simulink model "TFlex_FRF"  (R2018a)
settings: Solver=FixedStepDiscrete  StartTime=0.0  StopTime=t_end  FixedStep=0.001  RelTol=1e-3
PreLoadFcn:
  | Ts = 0.001;
InitFcn:
  | Ts = 0.001;
values from neighbouring files (symbols this model uses):
  t_end = 200    [Tflex_PID_init.m]    (also in multisineInit.m = t(end))
  ts = 1/1000    (= 0.001)    [Tflex_PID_init.m]    (also in init.m = 0.00025; multisineInit.m)
libraries: xpcethercatlib x91, simulink x60, slrtlib x6
(part 1 of 2)
settings Model: xpc_rtwmakecfg_data=_xpcethercatlib_  SimulationMode=external  ExtModeTrigDirection=either  ExplicitPartitioning=on  Creator=lab  LastModifiedBy=wout7
settings DataIOCC: Decimation=10  LimitDataPoints=on  SaveFormat=StructureWithTime
settings OptimizationCC: BlockReduction=off  OptimizeBlockIOStorage=off  BufferReuse=off  GlobalBufferReuse=off  ExpressionFolding=off  LocalBlockOutputs=off  OptimizeDataStoreBuffers=off  BusAssignmentInplaceUpdate=off
settings DebuggingCC: UnconnectedInputMsg=none  UnconnectedOutputMsg=none  UnconnectedLineMsg=none
settings HardwareCC: ProdBitPerPointer=32  ProdBitPerSizeT=32  ProdBitPerPtrDiffT=32  ProdLargestAtomicFloat=None  ProdWordSize=32  ProdLongLongMode=on  ProdHWDeviceType=Generic->32-bit x86 compatible
settings RTWCC: SystemTargetFile=slrt.tlc  TemplateMakefile=slrt_default_tmf  Description=Simulink Real-Time  CodeExecutionProfiling=on
settings SimulinkRealTimeCC: SupportVariableSizeSignals=on  xPCConcurrentTasks=on

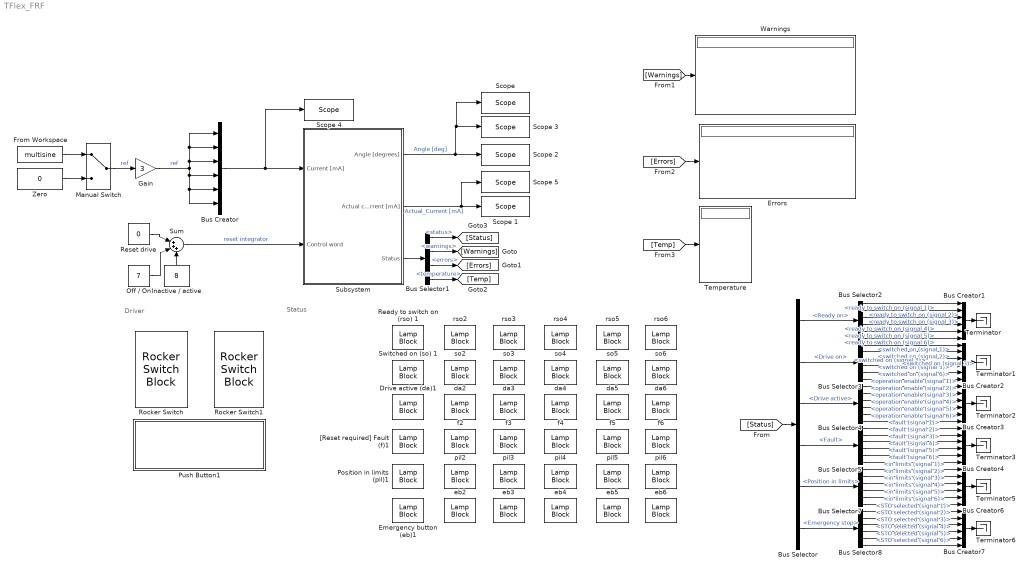
== system TFlex_FRF ==
  note: Driver
  note: Status
  " da2 " : LampBlock  WebBlockId=1372  LabelPosition=Hide
  " so2 " : LampBlock  WebBlockId=1336  LabelPosition=Hide
  " da4" : LampBlock  WebBlockId=1373  LabelPosition=Hide
  " da5" : LampBlock  WebBlockId=1374  LabelPosition=Hide
  " da6" : LampBlock  WebBlockId=1375  LabelPosition=Hide
  " eb4" : LampBlock  WebBlockId=1402  LabelPosition=Hide
  " eb5" : LampBlock  WebBlockId=1403  LabelPosition=Hide
  " eb6" : LampBlock  WebBlockId=1404  LabelPosition=Hide
  " f4" : LampBlock  WebBlockId=1379  LabelPosition=Hide
  " f5" : LampBlock  WebBlockId=1380  LabelPosition=Hide
  " f6" : LampBlock  WebBlockId=1381  LabelPosition=Hide
  " pil4" : LampBlock  WebBlockId=1397  LabelPosition=Hide
  " pil5" : LampBlock  WebBlockId=1398  LabelPosition=Hide
  " pil6" : LampBlock  WebBlockId=1399  LabelPosition=Hide
  " rso4" : LampBlock  WebBlockId=1325  LabelPosition=Hide
  " so4" : LampBlock  WebBlockId=1333  LabelPosition=Hide
  " so5" : LampBlock  WebBlockId=1334  LabelPosition=Hide
  " so6" : LampBlock  WebBlockId=1335  LabelPosition=Hide
  Bus Creator{,1..4,6..7} (7 alike) : BusCreator  Inputs=6
  Bus Selector : BusSelector  OutputSignals=Ready on,Drive on,Drive active,Fault,Position in limits,Emergency stop
  Bus Selector1 : BusSelector  OutputSignals=status,warnings,errors,temperature
  Bus Selector2 : BusSelector  OutputSignals=ready to switch on (signal 1),ready to switch on (signal 2),ready to switch on (signal 3),ready to switch on (signal 4),ready to switch on (signal 5),ready to switch on (signal 6)
  Bus Selector3 : BusSelector  OutputSignals=switched on (signal 1),switched on (signal 2),switched on (signal 3),switched on (signal 4),switched on (signal 5),switched on (signal 6)
  Bus Selector4 : BusSelector  OutputSignals=operation enable (signal 1),operation enable (signal 2),operation enable (signal 3),operation enable (signal 4),operation enable (signal 5),operation enable (signal 6)
  Bus Selector5 : BusSelector  OutputSignals=fault (signal 1),fault (signal 2),fault (signal 3),fault (signal 4),fault (signal 5),fault (signal 6)
  Bus Selector7 : BusSelector  OutputSignals=in limits (signal 1),in limits (signal 2),in limits (signal 3),in limits (signal 4),in limits (signal 5),in limits (signal 6)
  Bus Selector8 : BusSelector  OutputSignals=STO selected (signal 1),STO selected (signal 2),STO selected (signal 3),STO selected (signal 4),STO selected (signal 5),STO selected (signal 6)
  Drive active (da)1 : LampBlock  WebBlockId=1376
  Emergency button (eb)1 : LampBlock  WebBlockId=1405
  Errors : Display
      settings: Decimation=25
  From Workspace : FromWorkspace  VariableName=multisine  OutputAfterFinalValue=Setting to zero
  Gain : Gain  Gain=3
  Inactive / active : Constant  Value=8  SampleTime=-1
  Manual Switch : ManualSwitch
  Off / On : Constant  Value=7  SampleTime=-1
  Position in limits (pil)1 : LampBlock  WebBlockId=1400
  Push Button1 : Subsystem  DialogController=hmiCreateDDGDialog  IsWebBlock=on  mask(MWDashboardBlock){webBlockId=c834c18b-4d14-4fd2-a2aa-8470ccae1b8a, webBlockType=pushbutton, ShowInLibBrwoser=on, ShowInitialText=on, HMISrcModelName=TFlex_FRF}
      mask prompts: webBlockId "WebBlock Id"; webBlockType "WebBlock Type"; HMISrcModelName "Source Model"
      mask help: SimulinkHMI:dialogs:PushButtonDialogDesc
      mask Help: helpview([docroot '/mapfiles/simulink.map'], 'hmi_push_button')
      mask Display:
      | model = bdroot(gcb);
      | if strcmp(get_param(model,'BlockDiagramType'), 'library')
      |     image([(matlabroot) '/toolbox/simulink/hmi/icons/PushButton.png']);
      | end
  Ready to switch on (rso) 1 : LampBlock  WebBlockId=226
  Reset drive : Constant  Value=0  SampleTime=-1
  Rocker Switch : RockerSwitchBlock  WebBlockId=231
      settings: Values={{'Off', 'On'}, [6 7]}
  Rocker Switch1 : RockerSwitchBlock  WebBlockId=232
      settings: Values={{'Off', 'On'}, [0 8]}
  "Scope " : slrtlib/Displays and Logging/Scope   scopeno=4  scopetype=File  autostart=on  viewmode=Graphical redraw  formatstr='%15.6f'  grid=on  ylimits=[0,0]  nosamples=t_end/ts  noprepostsamples=0  interleave=1  triggermode=FreeRun  triggersignal=1  trigsignalfromport=off  triggerlevel=0.0  triggerslope=Either  triggerscope=1  triggersample=0  filename=ANGLE.dat  mode=Lazy  writesize=512  autorestart=off  dynamicfilemode=off  maxwritefilesize=512*1024^2
  Scope 1 : slrtlib/Displays and Logging/Scope   scopeno=2  scopetype=Target  autostart=on  viewmode=Graphical sliding  formatstr='%15.6f,%15.6f,%15.6f,%15.6f,%15.6f,%15.6f'  grid=on  ylimits=[-500,500]  nosamples=2000  noprepostsamples=0  interleave=25  triggermode=FreeRun  triggersignal=1  trigsignalfromport=off  triggerlevel=0.0  triggerslope=Either  triggerscope=1  triggersample=0  filename=data.dat  mode=Lazy  writesize=512  autorestart=off  dynamicfilemode=off  maxwritefilesize=512*1024^2
  Scope 2 : slrtlib/Displays and Logging/Scope   scopeno=1  scopetype=Target  autostart=on  viewmode=Numerical  formatstr='%15.6f,%15.6f,%15.6f,%15.6f,%15.6f,%15.6f'  grid=on  ylimits=[500,500]  nosamples=100  noprepostsamples=0  interleave=25  triggermode=FreeRun  triggersignal=1  trigsignalfromport=off  triggerlevel=0.0  triggerslope=Either  triggerscope=1  triggersample=0  filename=data.dat  mode=Lazy  writesize=512  autorestart=off  dynamicfilemode=off  maxwritefilesize=512*1024^2
  Scope 3 : slrtlib/Displays and Logging/Scope   scopeno=3  scopetype=Target  autostart=on  viewmode=Graphical sliding  formatstr='%15.6f,%15.6f,%15.6f,%15.6f,%15.6f,%15.6f'  grid=on  ylimits=[-20,20]  nosamples=3000  noprepostsamples=0  interleave=25  triggermode=FreeRun  triggersignal=1  trigsignalfromport=off  triggerlevel=0.0  triggerslope=Either  triggerscope=1  triggersample=0  filename=data.dat  mode=Lazy  writesize=512  autorestart=off  dynamicfilemode=off  maxwritefilesize=512*1024^2
  Scope 4 : slrtlib/Displays and Logging/Scope   scopeno=5  scopetype=File  autostart=on  viewmode=Graphical redraw  formatstr='%15.6f'  grid=on  ylimits=[0,0]  nosamples=t_end/ts  noprepostsamples=0  interleave=1  triggermode=FreeRun  triggersignal=1  trigsignalfromport=off  triggerlevel=0.0  triggerslope=Either  triggerscope=1  triggersample=0  filename=I_SP.dat  mode=Lazy  writesize=512  autorestart=off  dynamicfilemode=off  maxwritefilesize=512*1024^2
  Scope 5 : slrtlib/Displays and Logging/Scope   scopeno=6  scopetype=File  autostart=on  viewmode=Graphical redraw  formatstr='%15.6f'  grid=on  ylimits=[0,0]  nosamples=t_end/ts  noprepostsamples=0  interleave=1  triggermode=FreeRun  triggersignal=1  trigsignalfromport=off  triggerlevel=0.0  triggerslope=Either  triggerscope=1  triggersample=0  filename=I_A.dat  mode=Lazy  writesize=512  autorestart=off  dynamicfilemode=off  maxwritefilesize=512*1024^2
  Subsystem : Subsystem  TreatAsAtomicUnit=on
  Sum : Sum  Inputs=|+++
  Switched on (so) 1 : LampBlock  WebBlockId=1338
  Temperature : Display
      settings: Decimation=25
  Terminator{,1..3,5..6} (6 alike) : Terminator
  Warnings : Display
      settings: Decimation=25
  Zero : Constant  Value=0
  "[Reset required] Fault (f)1 " : LampBlock  WebBlockId=1382
  da3 : LampBlock  WebBlockId=1377  LabelPosition=Hide
  eb2 : LampBlock  WebBlockId=1406  LabelPosition=Hide
  eb3 : LampBlock  WebBlockId=1407  LabelPosition=Hide
  f2 : LampBlock  WebBlockId=1378  LabelPosition=Hide
  f3 : LampBlock  WebBlockId=1383  LabelPosition=Hide
  pil2 : LampBlock  WebBlockId=1396  LabelPosition=Hide
  pil3 : LampBlock  WebBlockId=1401  LabelPosition=Hide
  rso2 : LampBlock  WebBlockId=1323  LabelPosition=Hide
  rso3 : LampBlock  WebBlockId=1324  LabelPosition=Hide
  rso5 : LampBlock  WebBlockId=1326  LabelPosition=Hide
  rso6 : LampBlock  WebBlockId=1327  LabelPosition=Hide
  so3 : LampBlock  WebBlockId=1337  LabelPosition=Hide
  wires:
  Subsystem/2(Actual current [mA]) -> Scope 5/1, Scope 1/1  "Actual_Current [mA]"
  Bus Selector/1 -> Bus Selector2/1  "<Ready on>"
  Bus Selector/2 -> Bus Selector3/1  "<Drive on>"
  Bus Selector/3 -> Bus Selector4/1  "<Drive active>"
  Bus Selector/4 -> Bus Selector5/1  "<Fault>"
  Bus Selector/5 -> Bus Selector7/1  "<Position in limits>"
  Bus Selector/6 -> Bus Selector8/1  "<Emergency stop>"
  Reset drive/1 -> Sum/1
  Off / On/1 -> Sum/2
  Inactive / active/1 -> Sum/3
  Subsystem/1(Angle [degrees]) -> "Scope "/1, Scope 3/1, Scope 2/1  "Angle [deg]"
  Manual Switch/1 -> Gain/1  "ref"
  Subsystem/3(Status) -> Bus Selector1/1
  [Temp] -> Temperature/1
  [Errors] -> Errors/1
  [Warnings] -> Warnings/1
  [Status] -> Bus Selector/1
  Bus Selector2/1 -> Bus Creator1/1  "<ready to switch on (signal 1)>"
  Bus Selector2/2 -> Bus Creator1/2  "<ready to switch on (signal 2)>"
  Bus Selector2/3 -> Bus Creator1/3  "<ready to switch on (signal 3)>"
  Bus Selector2/4 -> Bus Creator1/4  "<ready to switch on (signal 4)>"
  Bus Selector2/5 -> Bus Creator1/5  "<ready to switch on (signal 5)>"
  Bus Selector2/6 -> Bus Creator1/6  "<ready to switch on (signal 6)>"
  Bus Creator1/1 -> Terminator/1
  Bus Selector3/2 -> Bus Creator2/2  "<switched on (signal 2)>"
  Bus Selector3/1 -> Bus Creator2/1  "<switched on (signal 1)>"
  Bus Selector3/5 -> Bus Creator2/5  "<switched on (signal 5)>"
  Bus Creator2/1 -> Terminator1/1
  Bus Selector3/4 -> Bus Creator2/4  "<switched on (signal 4)>"
  Bus Selector3/6 -> Bus Creator2/6  "<switched on (signal 6)>"
  Bus Selector3/3 -> Bus Creator2/3  "<switched on (signal 3)>"
  Bus Selector4/4 -> Bus Creator3/4  "<operation enable (signal 4)>"
  Bus Selector4/6 -> Bus Creator3/6  "<operation enable (signal 6)>"
  Bus Creator3/1 -> Terminator2/1
  Bus Selector4/5 -> Bus Creator3/5  "<operation enable (signal 5)>"
  Bus Selector4/1 -> Bus Creator3/1  "<operation enable (signal 1)>"
  Bus Selector4/2 -> Bus Creator3/2  "<operation enable (signal 2)>"
  Bus Selector4/3 -> Bus Creator3/3  "<operation enable (signal 3)>"
  Bus Selector5/4 -> Bus Creator4/4  "<fault (signal 4)>"
  Bus Selector5/6 -> Bus Creator4/6  "<fault (signal 6)>"
  Bus Creator4/1 -> Terminator3/1
  Bus Selector5/5 -> Bus Creator4/5  "<fault (signal 5)>"
  Bus Selector5/1 -> Bus Creator4/1  "<fault (signal 1)>"
  Bus Selector5/2 -> Bus Creator4/2  "<fault (signal 2)>"
  Bus Selector5/3 -> Bus Creator4/3  "<fault (signal 3)>"
  Bus Selector7/4 -> Bus Creator6/4  "<in limits (signal 4)>"
  Bus Selector7/6 -> Bus Creator6/6  "<in limits (signal 6)>"
  Bus Creator6/1 -> Terminator5/1
  Bus Selector7/5 -> Bus Creator6/5  "<in limits (signal 5)>"
  Bus Selector7/1 -> Bus Creator6/1  "<in limits (signal 1)>"
  Bus Selector7/2 -> Bus Creator6/2  "<in limits (signal 2)>"
  Bus Selector7/3 -> Bus Creator6/3  "<in limits (signal 3)>"
  Bus Selector8/4 -> Bus Creator7/4  "<STO selected (signal 4)>"
  Bus Selector8/6 -> Bus Creator7/6  "<STO selected (signal 6)>"
  Bus Creator7/1 -> Terminator6/1
  Bus Selector8/5 -> Bus Creator7/5  "<STO selected (signal 5)>"
  Bus Selector8/1 -> Bus Creator7/1  "<STO selected (signal 1)>"
  Bus Selector8/2 -> Bus Creator7/2  "<STO selected (signal 2)>"
  Bus Selector8/3 -> Bus Creator7/3  "<STO selected (signal 3)>"
  Bus Creator/1 -> Scope 4/1, Subsystem/1(Current [mA])
  Sum/1 -> Subsystem/2(Control word)  "reset integrator"
  Bus Selector1/1 -> [Status]  "<status>"
  Bus Selector1/2 -> [Warnings]  "<warnings>"
  Bus Selector1/3 -> [Errors]  "<errors>"
  Bus Selector1/4 -> [Temp]  "<temperature>"
  From Workspace/1 -> Manual Switch/1
  Zero/1 -> Manual Switch/2
  Gain/1 -> Bus Creator/4, Bus Creator/5, Bus Creator/6, Bus Creator/3, Bus Creator/2, Bus Creator/1  "ref"

== system TFlex_FRF/Push Button1 ==

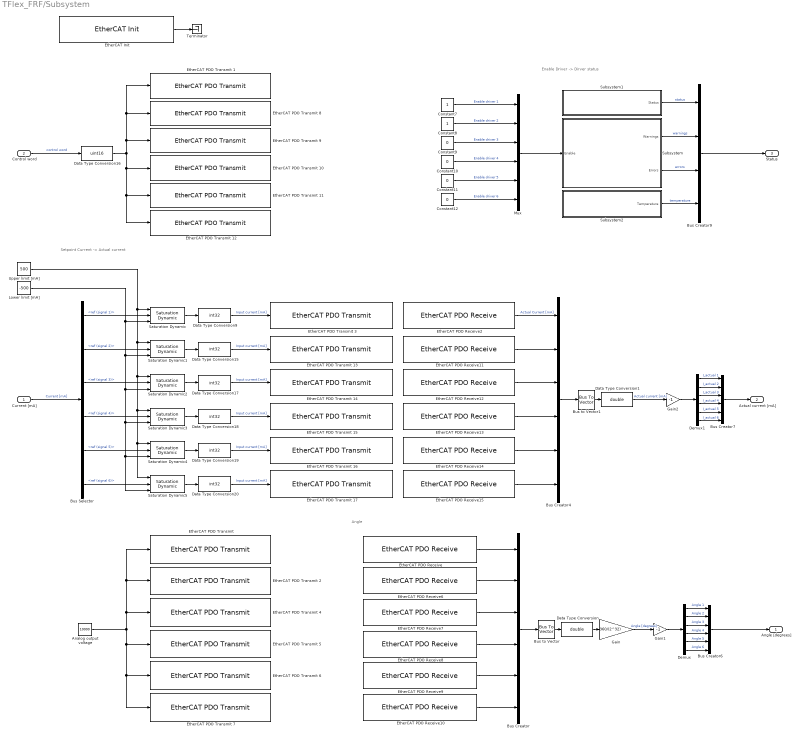
== system TFlex_FRF/Subsystem ==
  note: Angle
  note: Enable Driver -> Dirver status
  note: Setpoint Current -> Actual current
  Current [mA] : Inport  PortDimensions=6
  Control word : Inport  Port=2
  Analog output voltage : Constant  Value=10000  OutDataTypeStr=int16  SampleTime=-1
  Bus Creator{,4,6..7} (4 alike) : BusCreator  Inputs=6
  Bus Creator9 : BusCreator  Inputs=4
  Bus Selector : BusSelector  OutputSignals=ref (signal 1),ref (signal 2),ref (signal 3),ref (signal 4),ref (signal 5),ref (signal 6)
  Bus to Vector : BusToVector
  Bus to Vector1 : BusToVector
  Constant{9..12} (4 alike) : Constant  Value=0  OutDataTypeStr=int32  SampleTime=1
  Constant7 : Constant  OutDataTypeStr=int32  SampleTime=1
  Constant8 : Constant  OutDataTypeStr=int32  SampleTime=1
  Data Type Conversion : DataTypeConversion  OutDataTypeStr=double
  Data Type Conversion1 : DataTypeConversion  OutDataTypeStr=double
  Data Type Conversion{9,15,17..20} (6 alike) : DataTypeConversion  OutDataTypeStr=int32
  Data Type Conversion16 : DataTypeConversion  OutDataTypeStr=uint16
  Demux : Demux  Outputs=6
  Demux1 : Demux  Outputs=6
  "EtherCAT Init " : xpcethercatlib/EtherCAT Init   Priority=0  config_file=C:\Users\wout7\Documents\GitHub\Inverse_dynamics_learning\TargetPC\6 DOF\pdo_mapping_6dr_1kHz.xml  device_id=0  pci_bus=13  pci_slot=0  pci_function=0  dctuning=0  enaDebug=off  enaDC=on  errLink=off  masterDbg=off  stateChgDbg=off  baseClock=off  masterCfg=off  logFile='c:\dbglog.txt'  sample_time=0.001000  DCMode=2
      settings: SourceProductName=Simulink Real-Time  SourceProductBaseCode=XP
  EtherCAT PDO Receive : xpcethercatlib/EtherCAT PDO Receive  Priority=2  sig_name=Drive 2 (AKD).Inputs_1.Position actual internal value  sig_offset=560  sig_type=int32  type_size=32  sig_dim=1  device_id=0  sample_time=0.001000
      settings: SourceProductName=Simulink Real-Time  SourceProductBaseCode=XP
  EtherCAT PDO Receive10 : xpcethercatlib/EtherCAT PDO Receive  Priority=2  sig_name=Drive 7 (AKD).Inputs_1.Position actual internal value  sig_offset=37488  sig_type=int32  type_size=32  sig_dim=1  device_id=0  sample_time=0.001000
      settings: SourceProductName=Simulink Real-Time  SourceProductBaseCode=XP
  EtherCAT PDO Receive11 : xpcethercatlib/EtherCAT PDO Receive  Priority=2  sig_name=Drive 3 (AKD).Inputs_1.Current actual value  sig_offset=12560  sig_type=int32  type_size=32  sig_dim=1  device_id=0  sample_time=0.001000
      settings: SourceProductName=Simulink Real-Time  SourceProductBaseCode=XP
  EtherCAT PDO Receive12 : xpcethercatlib/EtherCAT PDO Receive  Priority=2  sig_name=Drive 4 (AKD).Inputs_1.Current actual value  sig_offset=24848  sig_type=int32  type_size=32  sig_dim=1  device_id=0  sample_time=0.001000
      settings: SourceProductName=Simulink Real-Time  SourceProductBaseCode=XP
  EtherCAT PDO Receive13 : xpcethercatlib/EtherCAT PDO Receive  Priority=2  sig_name=Drive 5 (AKD).Inputs_1.Current actual value  sig_offset=37136  sig_type=int32  type_size=32  sig_dim=1  device_id=0  sample_time=0.001000
      settings: SourceProductName=Simulink Real-Time  SourceProductBaseCode=XP
  EtherCAT PDO Receive14 : xpcethercatlib/EtherCAT PDO Receive  Priority=2  sig_name=Drive 6 (AKD).Inputs_1.Current actual value  sig_offset=37296  sig_type=int32  type_size=32  sig_dim=1  device_id=0  sample_time=0.001000
      settings: SourceProductName=Simulink Real-Time  SourceProductBaseCode=XP
  EtherCAT PDO Receive15 : xpcethercatlib/EtherCAT PDO Receive  Priority=2  sig_name=Drive 7 (AKD).Inputs_1.Current actual value  sig_offset=37456  sig_type=int32  type_size=32  sig_dim=1  device_id=0  sample_time=0.001000
      settings: SourceProductName=Simulink Real-Time  SourceProductBaseCode=XP
  EtherCAT PDO Receive2 : xpcethercatlib/EtherCAT PDO Receive  Priority=2  sig_name=Drive 2 (AKD).Inputs_1.Current actual value  sig_offset=528  sig_type=int32  type_size=32  sig_dim=1  device_id=0  sample_time=0.001000
      settings: SourceProductName=Simulink Real-Time  SourceProductBaseCode=XP
  EtherCAT PDO Receive6 : xpcethercatlib/EtherCAT PDO Receive  Priority=2  sig_name=Drive 3 (AKD).Inputs_1.Position actual internal value  sig_offset=12592  sig_type=int32  type_size=32  sig_dim=1  device_id=0  sample_time=0.001000
      settings: SourceProductName=Simulink Real-Time  SourceProductBaseCode=XP
  EtherCAT PDO Receive7 : xpcethercatlib/EtherCAT PDO Receive  Priority=2  sig_name=Drive 4 (AKD).Inputs_1.Position actual internal value  sig_offset=24880  sig_type=int32  type_size=32  sig_dim=1  device_id=0  sample_time=0.001000
      settings: SourceProductName=Simulink Real-Time  SourceProductBaseCode=XP
  EtherCAT PDO Receive8 : xpcethercatlib/EtherCAT PDO Receive  Priority=2  sig_name=Drive 5 (AKD).Inputs_1.Position actual internal value  sig_offset=37168  sig_type=int32  type_size=32  sig_dim=1  device_id=0  sample_time=0.001000
      settings: SourceProductName=Simulink Real-Time  SourceProductBaseCode=XP
  EtherCAT PDO Receive9 : xpcethercatlib/EtherCAT PDO Receive  Priority=2  sig_name=Drive 6 (AKD).Inputs_1.Position actual internal value  sig_offset=37328  sig_type=int32  type_size=32  sig_dim=1  device_id=0  sample_time=0.001000
      settings: SourceProductName=Simulink Real-Time  SourceProductBaseCode=XP
  "EtherCAT PDO Transmit " : xpcethercatlib/EtherCAT PDO Transmit   Priority=3  sig_name=Drive 2 (AKD).Outputs.AOUT.VALUE write  sig_offset=480  sig_type=int16  type_size=16  sig_dim=1  device_id=0  sample_time=0.001000
      settings: SourceProductName=Simulink Real-Time  SourceProductBaseCode=XP
  EtherCAT PDO Transmit 1 : xpcethercatlib/EtherCAT PDO Transmit   Priority=3  sig_name=Drive 2 (AKD).Outputs.Controlword  sig_offset=464  sig_type=uint16  type_size=16  sig_dim=1  device_id=0  sample_time=0.001000
      settings: SourceProductName=Simulink Real-Time  SourceProductBaseCode=XP
  EtherCAT PDO Transmit 10 : xpcethercatlib/EtherCAT PDO Transmit   Priority=3  sig_name=Drive 5 (AKD).Outputs.Controlword  sig_offset=37072  sig_type=uint16  type_size=16  sig_dim=1  device_id=0  sample_time=0.001000
      settings: SourceProductName=Simulink Real-Time  SourceProductBaseCode=XP
  EtherCAT PDO Transmit 11 : xpcethercatlib/EtherCAT PDO Transmit   Priority=3  sig_name=Drive 6 (AKD).Outputs.Controlword  sig_offset=37232  sig_type=uint16  type_size=16  sig_dim=1  device_id=0  sample_time=0.001000
      settings: SourceProductName=Simulink Real-Time  SourceProductBaseCode=XP
  EtherCAT PDO Transmit 12 : xpcethercatlib/EtherCAT PDO Transmit   Priority=3  sig_name=Drive 7 (AKD).Outputs.Controlword  sig_offset=37392  sig_type=uint16  type_size=16  sig_dim=1  device_id=0  sample_time=0.001000
      settings: SourceProductName=Simulink Real-Time  SourceProductBaseCode=XP
  EtherCAT PDO Transmit 13 : xpcethercatlib/EtherCAT PDO Transmit   Priority=3  sig_name=Drive 3 (AKD).Outputs.Target current  sig_offset=12528  sig_type=int32  type_size=32  sig_dim=1  device_id=0  sample_time=0.001000
      settings: SourceProductName=Simulink Real-Time  SourceProductBaseCode=XP
  EtherCAT PDO Transmit 14 : xpcethercatlib/EtherCAT PDO Transmit   Priority=3  sig_name=Drive 4 (AKD).Outputs.Target current  sig_offset=24816  sig_type=int32  type_size=32  sig_dim=1  device_id=0  sample_time=0.001000
      settings: SourceProductName=Simulink Real-Time  SourceProductBaseCode=XP
  EtherCAT PDO Transmit 15 : xpcethercatlib/EtherCAT PDO Transmit   Priority=3  sig_name=Drive 5 (AKD).Outputs.Target current  sig_offset=37104  sig_type=int32  type_size=32  sig_dim=1  device_id=0  sample_time=0.001000
      settings: SourceProductName=Simulink Real-Time  SourceProductBaseCode=XP
  EtherCAT PDO Transmit 16 : xpcethercatlib/EtherCAT PDO Transmit   Priority=3  sig_name=Drive 6 (AKD).Outputs.Target current  sig_offset=37264  sig_type=int32  type_size=32  sig_dim=1  device_id=0  sample_time=0.001000
      settings: SourceProductName=Simulink Real-Time  SourceProductBaseCode=XP
  EtherCAT PDO Transmit 17 : xpcethercatlib/EtherCAT PDO Transmit   Priority=3  sig_name=Drive 7 (AKD).Outputs.Target current  sig_offset=37424  sig_type=int32  type_size=32  sig_dim=1  device_id=0  sample_time=0.001000
      settings: SourceProductName=Simulink Real-Time  SourceProductBaseCode=XP
  EtherCAT PDO Transmit 2 : xpcethercatlib/EtherCAT PDO Transmit   Priority=3  sig_name=Drive 3 (AKD).Outputs.AOUT.VALUE write  sig_offset=12512  sig_type=int16  type_size=16  sig_dim=1  device_id=0  sample_time=0.001000
      settings: SourceProductName=Simulink Real-Time  SourceProductBaseCode=XP
  EtherCAT PDO Transmit 3 : xpcethercatlib/EtherCAT PDO Transmit   Priority=3  sig_name=Drive 2 (AKD).Outputs.Target current  sig_offset=496  sig_type=int32  type_size=32  sig_dim=1  device_id=0  sample_time=0.001000
      settings: SourceProductName=Simulink Real-Time  SourceProductBaseCode=XP
  EtherCAT PDO Transmit 4 : xpcethercatlib/EtherCAT PDO Transmit   Priority=3  sig_name=Drive 4 (AKD).Outputs.AOUT.VALUE write  sig_offset=24800  sig_type=int16  type_size=16  sig_dim=1  device_id=0  sample_time=0.001000
      settings: SourceProductName=Simulink Real-Time  SourceProductBaseCode=XP
  EtherCAT PDO Transmit 5 : xpcethercatlib/EtherCAT PDO Transmit   Priority=3  sig_name=Drive 5 (AKD).Outputs.AOUT.VALUE write  sig_offset=37088  sig_type=int16  type_size=16  sig_dim=1  device_id=0  sample_time=0.001000
      settings: SourceProductName=Simulink Real-Time  SourceProductBaseCode=XP
  EtherCAT PDO Transmit 6 : xpcethercatlib/EtherCAT PDO Transmit   Priority=3  sig_name=Drive 6 (AKD).Outputs.AOUT.VALUE write  sig_offset=37248  sig_type=int16  type_size=16  sig_dim=1  device_id=0  sample_time=0.001000
      settings: SourceProductName=Simulink Real-Time  SourceProductBaseCode=XP
  EtherCAT PDO Transmit 7 : xpcethercatlib/EtherCAT PDO Transmit   Priority=3  sig_name=Drive 7 (AKD).Outputs.AOUT.VALUE write  sig_offset=37408  sig_type=int16  type_size=16  sig_dim=1  device_id=0  sample_time=0.001000
      settings: SourceProductName=Simulink Real-Time  SourceProductBaseCode=XP
  EtherCAT PDO Transmit 8 : xpcethercatlib/EtherCAT PDO Transmit   Priority=3  sig_name=Drive 3 (AKD).Outputs.Controlword  sig_offset=12496  sig_type=uint16  type_size=16  sig_dim=1  device_id=0  sample_time=0.001000
      settings: SourceProductName=Simulink Real-Time  SourceProductBaseCode=XP
  EtherCAT PDO Transmit 9 : xpcethercatlib/EtherCAT PDO Transmit   Priority=3  sig_name=Drive 4 (AKD).Outputs.Controlword  sig_offset=24784  sig_type=uint16  type_size=16  sig_dim=1  device_id=0  sample_time=0.001000
      settings: SourceProductName=Simulink Real-Time  SourceProductBaseCode=XP
  Gain : Gain  Gain=360/(2^32)
  Gain1 : Gain  Gain=-1
  Gain2 : Gain  Gain=-1
  Lower limit [mA] : Constant  Value=-500
  Mux : Mux  Inputs=6
  Saturation Dynamic{,1..5} (6 alike) : simulink/Discontinuities/Saturation Dynamic  OutMin=[]  OutMax=[]  OutDataTypeStr=Inherit: Same as second input  OutDataType=fixdt(1, 16)  OutScaling=2^-10  DoSatur=off
  Subsystem : Subsystem
  Subsystem1 : Subsystem
  Subsystem2 : Subsystem
  Terminator : Terminator
  Upper limit [mA] : Constant  Value=500
  Angle [degrees] : Outport
  Actual current [mA] : Outport  Port=2
  Status : Outport  Port=3
  wires:
  EtherCAT PDO Receive12/1 -> Bus Creator4/3
  Upper limit [mA]/1 -> Saturation Dynamic3/1, Saturation Dynamic4/1, Saturation Dynamic5/1, Saturation Dynamic2/1, Saturation Dynamic1/1, Saturation Dynamic/1
  Bus Selector/1 -> Saturation Dynamic/2  "<ref (signal 1)>"
  Analog output voltage/1 -> EtherCAT PDO Transmit 7/1, EtherCAT PDO Transmit 6/1, EtherCAT PDO Transmit 5/1, "EtherCAT PDO Transmit "/1, EtherCAT PDO Transmit 2/1, EtherCAT PDO Transmit 4/1
  Bus Selector/4 -> Saturation Dynamic3/2  "<ref (signal 4)>"
  Saturation Dynamic/1 -> Data Type Conversion9/1
  Bus to Vector1/1 -> Data Type Conversion1/1
  EtherCAT PDO Receive2/1 -> Bus Creator4/1  "Actual Current [mA]"
  EtherCAT PDO Receive6/1 -> Bus Creator/2
  Saturation Dynamic5/1 -> Data Type Conversion20/1
  EtherCAT PDO Receive10/1 -> Bus Creator/6
  Data Type Conversion20/1 -> EtherCAT PDO Transmit 17/1  "Input current [mA]"
  Bus Selector/3 -> Saturation Dynamic2/2  "<ref (signal 3)>"
  EtherCAT PDO Receive9/1 -> Bus Creator/5
  Saturation Dynamic4/1 -> Data Type Conversion19/1
  Bus Selector/2 -> Saturation Dynamic1/2  "<ref (signal 2)>"
  EtherCAT PDO Receive7/1 -> Bus Creator/3
  Data Type Conversion/1 -> Gain/1
  Gain/1 -> Gain1/1  "Angle [degrees]"
  Demux/6 -> Bus Creator6/6  "Angle 6"
  Current [mA]/1 -> Bus Selector/1  "Current [mA]"
  Control word/1 -> Data Type Conversion16/1  "control word"
  Demux/3 -> Bus Creator6/3  "Angle 3"
  Bus Creator9/1 -> Status/1
  Saturation Dynamic3/1 -> Data Type Conversion18/1
  Data Type Conversion18/1 -> EtherCAT PDO Transmit 15/1  "Input current [mA]"
  Demux1/3 -> Bus Creator7/3  "I_actual 3"
  Bus Creator4/1 -> Bus to Vector1/1
  Data Type Conversion17/1 -> EtherCAT PDO Transmit 14/1  "Input current [mA]"
  Saturation Dynamic1/1 -> Data Type Conversion15/1
  Demux1/2 -> Bus Creator7/2  "I_actual 2"
  Demux/4 -> Bus Creator6/4  "Angle 4"
  Bus Selector/5 -> Saturation Dynamic4/2  "<ref (signal 5)>"
  Data Type Conversion16/1 -> EtherCAT PDO Transmit 1/1, EtherCAT PDO Transmit 8/1, EtherCAT PDO Transmit 9/1, EtherCAT PDO Transmit 12/1, EtherCAT PDO Transmit 11/1, EtherCAT PDO Transmit 10/1
  EtherCAT PDO Receive/1 -> Bus Creator/1
  EtherCAT PDO Receive15/1 -> Bus Creator4/6
  Data Type Conversion15/1 -> EtherCAT PDO Transmit 13/1  "Input current [mA]"
  Bus to Vector/1 -> Data Type Conversion/1
  Data Type Conversion19/1 -> EtherCAT PDO Transmit 16/1  "Input current [mA]"
  Demux/1 -> Bus Creator6/1  "Angle 1"
  Lower limit [mA]/1 -> Saturation Dynamic/3, Saturation Dynamic1/3, Saturation Dynamic2/3, Saturation Dynamic3/3, Saturation Dynamic4/3, Saturation Dynamic5/3
  EtherCAT PDO Receive13/1 -> Bus Creator4/4
  "EtherCAT Init "/1 -> Terminator/1
  Data Type Conversion1/1 -> Gain2/1  "Actual current [mA]"
  Demux/5 -> Bus Creator6/5  "Angle 5"
  Demux1/4 -> Bus Creator7/4  "I_actual 4"
  Demux1/6 -> Bus Creator7/6  "I_actual 6"
  Bus Creator/1 -> Bus to Vector/1
  EtherCAT PDO Receive11/1 -> Bus Creator4/2
  Bus Selector/6 -> Saturation Dynamic5/2  "<ref (signal 6)>"
  EtherCAT PDO Receive14/1 -> Bus Creator4/5
  Data Type Conversion9/1 -> EtherCAT PDO Transmit 3/1  "Input current [mA]"
  EtherCAT PDO Receive8/1 -> Bus Creator/4
  Demux1/1 -> Bus Creator7/1  "I_actual 1"
  Demux1/5 -> Bus Creator7/5  "I_actual 5"
  Demux/2 -> Bus Creator6/2  "Angle 2"
  Bus Creator6/1 -> Angle [degrees]/1
  Saturation Dynamic2/1 -> Data Type Conversion17/1
  Bus Creator7/1 -> Actual current [mA]/1
  Constant7/1 -> Mux/1  "Enable driver 1"
  Constant8/1 -> Mux/2  "Enable driver 2"
  Constant9/1 -> Mux/3  "Enable driver 3"
  Constant10/1 -> Mux/4  "Enable driver 4"
  Constant11/1 -> Mux/5  "Enable driver 5"
  Constant12/1 -> Mux/6  "Enable driver 6"
  Mux/1 -> Subsystem/1(Enable)
  Subsystem/1(Warnings) -> Bus Creator9/2  "warnings"
  Subsystem/2(Errors) -> Bus Creator9/3  "errors"
  Subsystem1/1(Status) -> Bus Creator9/1  "status"
  Subsystem2/1(Temperature) -> Bus Creator9/4  "temperature"
  Gain1/1 -> Demux/1
  Gain2/1 -> Demux1/1

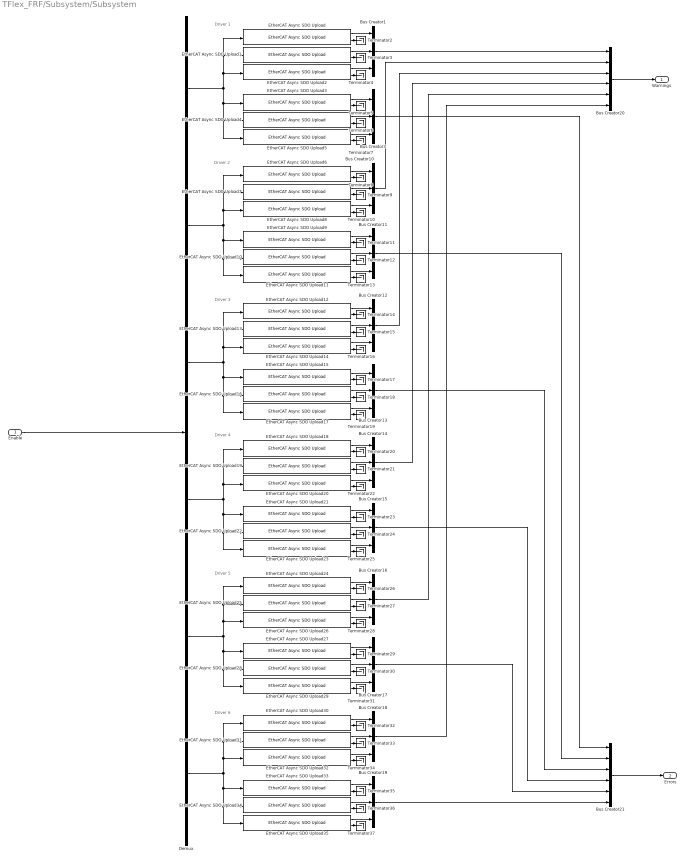
== system TFlex_FRF/Subsystem/Subsystem ==
  note: Driver 1
  note: Driver 2
  note: Driver 3
  note: Driver 4
  note: Driver 5
  note: Driver 6
  Enable : Inport
  Bus Creator{1,3,10..19} (12 alike) : BusCreator  Inputs=3
  Bus Creator20 : BusCreator  Inputs=6
  Bus Creator21 : BusCreator  Inputs=6
  Demux : Demux  Outputs=6
  EtherCAT Async SDO Upload : xpcethercatlib/EtherCAT Async SDO Upload  index=8192  subIndex=1  sig_type=uint32  sig_dim=1  device_id=0  slave_name=Drive 2 (AKD)  sample_time=1  slave_addr=1001  selected_slave=Term 1 (EK1100)  timeout=500  slave_found=1
      settings: SourceProductName=Simulink Real-Time  SourceProductBaseCode=XP
  EtherCAT Async SDO Upload1 : xpcethercatlib/EtherCAT Async SDO Upload  index=8192  subIndex=2  sig_type=uint32  sig_dim=1  device_id=0  slave_name=Drive 2 (AKD)  sample_time=1  slave_addr=1001  selected_slave=Term 1 (EK1100)  timeout=500  slave_found=1
      settings: SourceProductName=Simulink Real-Time  SourceProductBaseCode=XP
  EtherCAT Async SDO Upload10 : xpcethercatlib/EtherCAT Async SDO Upload  index=8193  subIndex=2  sig_type=uint32  sig_dim=1  device_id=0  slave_name=Drive 3 (AKD)  sample_time=1  slave_addr=1002  selected_slave=Term 1 (EK1100)  timeout=500  slave_found=1
      settings: SourceProductName=Simulink Real-Time  SourceProductBaseCode=XP
  EtherCAT Async SDO Upload11 : xpcethercatlib/EtherCAT Async SDO Upload  index=8193  subIndex=3  sig_type=uint32  sig_dim=1  device_id=0  slave_name=Drive 3 (AKD)  sample_time=1  slave_addr=1002  selected_slave=Term 1 (EK1100)  timeout=500  slave_found=1
      settings: SourceProductName=Simulink Real-Time  SourceProductBaseCode=XP
  EtherCAT Async SDO Upload12 : xpcethercatlib/EtherCAT Async SDO Upload  index=8192  subIndex=1  sig_type=uint32  sig_dim=1  device_id=0  slave_name=Drive 4 (AKD)  sample_time=1  slave_addr=1003  selected_slave=Term 1 (EK1100)  timeout=500  slave_found=1
      settings: SourceProductName=Simulink Real-Time  SourceProductBaseCode=XP
  EtherCAT Async SDO Upload13 : xpcethercatlib/EtherCAT Async SDO Upload  index=8192  subIndex=2  sig_type=uint32  sig_dim=1  device_id=0  slave_name=Drive 4 (AKD)  sample_time=1  slave_addr=1003  selected_slave=Term 1 (EK1100)  timeout=500  slave_found=1
      settings: SourceProductName=Simulink Real-Time  SourceProductBaseCode=XP
  EtherCAT Async SDO Upload14 : xpcethercatlib/EtherCAT Async SDO Upload  index=8192  subIndex=3  sig_type=uint32  sig_dim=1  device_id=0  slave_name=Drive 4 (AKD)  sample_time=1  slave_addr=1003  selected_slave=Term 1 (EK1100)  timeout=500  slave_found=1
      settings: SourceProductName=Simulink Real-Time  SourceProductBaseCode=XP
  EtherCAT Async SDO Upload15 : xpcethercatlib/EtherCAT Async SDO Upload  index=8193  subIndex=1  sig_type=uint32  sig_dim=1  device_id=0  slave_name=Drive 4 (AKD)  sample_time=1  slave_addr=1003  selected_slave=Term 1 (EK1100)  timeout=500  slave_found=1
      settings: SourceProductName=Simulink Real-Time  SourceProductBaseCode=XP
  EtherCAT Async SDO Upload16 : xpcethercatlib/EtherCAT Async SDO Upload  index=8193  subIndex=2  sig_type=uint32  sig_dim=1  device_id=0  slave_name=Drive 4 (AKD)  sample_time=1  slave_addr=1003  selected_slave=Term 1 (EK1100)  timeout=500  slave_found=1
      settings: SourceProductName=Simulink Real-Time  SourceProductBaseCode=XP
  EtherCAT Async SDO Upload17 : xpcethercatlib/EtherCAT Async SDO Upload  index=8193  subIndex=3  sig_type=uint32  sig_dim=1  device_id=0  slave_name=Drive 4 (AKD)  sample_time=1  slave_addr=1003  selected_slave=Term 1 (EK1100)  timeout=500  slave_found=1
      settings: SourceProductName=Simulink Real-Time  SourceProductBaseCode=XP
  EtherCAT Async SDO Upload18 : xpcethercatlib/EtherCAT Async SDO Upload  index=8192  subIndex=1  sig_type=uint32  sig_dim=1  device_id=0  slave_name=Drive 5 (AKD)  sample_time=1  slave_addr=1004  selected_slave=Term 1 (EK1100)  timeout=500  slave_found=1
      settings: SourceProductName=Simulink Real-Time  SourceProductBaseCode=XP
  EtherCAT Async SDO Upload19 : xpcethercatlib/EtherCAT Async SDO Upload  index=8192  subIndex=2  sig_type=uint32  sig_dim=1  device_id=0  slave_name=Drive 5 (AKD)  sample_time=1  slave_addr=1004  selected_slave=Term 1 (EK1100)  timeout=500  slave_found=1
      settings: SourceProductName=Simulink Real-Time  SourceProductBaseCode=XP
  EtherCAT Async SDO Upload2 : xpcethercatlib/EtherCAT Async SDO Upload  index=8192  subIndex=3  sig_type=uint32  sig_dim=1  device_id=0  slave_name=Drive 1 (AKD)  sample_time=1  slave_addr=1001  selected_slave=Term 1 (EK1100)  timeout=500  slave_found=1
      settings: SourceProductName=Simulink Real-Time  SourceProductBaseCode=XP
  EtherCAT Async SDO Upload20 : xpcethercatlib/EtherCAT Async SDO Upload  index=8192  subIndex=3  sig_type=uint32  sig_dim=1  device_id=0  slave_name=Drive 5 (AKD)  sample_time=1  slave_addr=1004  selected_slave=Term 1 (EK1100)  timeout=500  slave_found=1
      settings: SourceProductName=Simulink Real-Time  SourceProductBaseCode=XP
  EtherCAT Async SDO Upload21 : xpcethercatlib/EtherCAT Async SDO Upload  index=8193  subIndex=1  sig_type=uint32  sig_dim=1  device_id=0  slave_name=Drive 5 (AKD)  sample_time=1  slave_addr=1004  selected_slave=Term 1 (EK1100)  timeout=500  slave_found=1
      settings: SourceProductName=Simulink Real-Time  SourceProductBaseCode=XP
  EtherCAT Async SDO Upload22 : xpcethercatlib/EtherCAT Async SDO Upload  index=8193  subIndex=2  sig_type=uint32  sig_dim=1  device_id=0  slave_name=Drive 5 (AKD)  sample_time=1  slave_addr=1004  selected_slave=Term 1 (EK1100)  timeout=500  slave_found=1
      settings: SourceProductName=Simulink Real-Time  SourceProductBaseCode=XP
  EtherCAT Async SDO Upload23 : xpcethercatlib/EtherCAT Async SDO Upload  index=8193  subIndex=3  sig_type=uint32  sig_dim=1  device_id=0  slave_name=Drive 5 (AKD)  sample_time=1  slave_addr=1004  selected_slave=Term 1 (EK1100)  timeout=500  slave_found=1
      settings: SourceProductName=Simulink Real-Time  SourceProductBaseCode=XP
  EtherCAT Async SDO Upload24 : xpcethercatlib/EtherCAT Async SDO Upload  index=8192  subIndex=1  sig_type=uint32  sig_dim=1  device_id=0  slave_name=Drive 6 (AKD)  sample_time=1  slave_addr=1005  selected_slave=Term 1 (EK1100)  timeout=500  slave_found=1
      settings: SourceProductName=Simulink Real-Time  SourceProductBaseCode=XP
  EtherCAT Async SDO Upload25 : xpcethercatlib/EtherCAT Async SDO Upload  index=8192  subIndex=2  sig_type=uint32  sig_dim=1  device_id=0  slave_name=Drive 6 (AKD)  sample_time=1  slave_addr=1005  selected_slave=Term 1 (EK1100)  timeout=500  slave_found=1
      settings: SourceProductName=Simulink Real-Time  SourceProductBaseCode=XP
  EtherCAT Async SDO Upload26 : xpcethercatlib/EtherCAT Async SDO Upload  index=8192  subIndex=3  sig_type=uint32  sig_dim=1  device_id=0  slave_name=Drive 6 (AKD)  sample_time=1  slave_addr=1005  selected_slave=Term 1 (EK1100)  timeout=500  slave_found=1
      settings: SourceProductName=Simulink Real-Time  SourceProductBaseCode=XP
  EtherCAT Async SDO Upload27 : xpcethercatlib/EtherCAT Async SDO Upload  index=8193  subIndex=1  sig_type=uint32  sig_dim=1  device_id=0  slave_name=Drive 6 (AKD)  sample_time=1  slave_addr=1005  selected_slave=Term 1 (EK1100)  timeout=500  slave_found=1
      settings: SourceProductName=Simulink Real-Time  SourceProductBaseCode=XP
  EtherCAT Async SDO Upload28 : xpcethercatlib/EtherCAT Async SDO Upload  index=8193  subIndex=2  sig_type=uint32  sig_dim=1  device_id=0  slave_name=Drive 6 (AKD)  sample_time=1  slave_addr=1005  selected_slave=Term 1 (EK1100)  timeout=500  slave_found=1
      settings: SourceProductName=Simulink Real-Time  SourceProductBaseCode=XP
  EtherCAT Async SDO Upload29 : xpcethercatlib/EtherCAT Async SDO Upload  index=8193  subIndex=3  sig_type=uint32  sig_dim=1  device_id=0  slave_name=Drive 6 (AKD)  sample_time=1  slave_addr=1005  selected_slave=Term 1 (EK1100)  timeout=500  slave_found=1
      settings: SourceProductName=Simulink Real-Time  SourceProductBaseCode=XP
  EtherCAT Async SDO Upload3 : xpcethercatlib/EtherCAT Async SDO Upload  index=8193  subIndex=1  sig_type=uint32  sig_dim=1  device_id=0  slave_name=""  sample_time=1  slave_addr=0  selected_slave=Term 1 (EK1100)  timeout=500  slave_found=1
      settings: SourceProductName=Simulink Real-Time  SourceProductBaseCode=XP
  EtherCAT Async SDO Upload30 : xpcethercatlib/EtherCAT Async SDO Upload  index=8192  subIndex=1  sig_type=uint32  sig_dim=1  device_id=0  slave_name=Drive 7 (AKD)  sample_time=1  slave_addr=1006  selected_slave=Term 1 (EK1100)  timeout=500  slave_found=1
      settings: SourceProductName=Simulink Real-Time  SourceProductBaseCode=XP
  EtherCAT Async SDO Upload31 : xpcethercatlib/EtherCAT Async SDO Upload  index=8192  subIndex=2  sig_type=uint32  sig_dim=1  device_id=0  slave_name=Drive 7 (AKD)  sample_time=1  slave_addr=1006  selected_slave=Term 1 (EK1100)  timeout=500  slave_found=1
      settings: SourceProductName=Simulink Real-Time  SourceProductBaseCode=XP
  EtherCAT Async SDO Upload32 : xpcethercatlib/EtherCAT Async SDO Upload  index=8192  subIndex=3  sig_type=uint32  sig_dim=1  device_id=0  slave_name=Drive 7 (AKD)  sample_time=1  slave_addr=1006  selected_slave=Term 1 (EK1100)  timeout=500  slave_found=1
      settings: SourceProductName=Simulink Real-Time  SourceProductBaseCode=XP
  EtherCAT Async SDO Upload33 : xpcethercatlib/EtherCAT Async SDO Upload  index=8193  subIndex=1  sig_type=uint32  sig_dim=1  device_id=0  slave_name=Drive 7 (AKD)  sample_time=1  slave_addr=1006  selected_slave=Term 1 (EK1100)  timeout=500  slave_found=1
      settings: SourceProductName=Simulink Real-Time  SourceProductBaseCode=XP
  EtherCAT Async SDO Upload34 : xpcethercatlib/EtherCAT Async SDO Upload  index=8193  subIndex=2  sig_type=uint32  sig_dim=1  device_id=0  slave_name=Drive 7 (AKD)  sample_time=1  slave_addr=1006  selected_slave=Term 1 (EK1100)  timeout=500  slave_found=1
      settings: SourceProductName=Simulink Real-Time  SourceProductBaseCode=XP
  EtherCAT Async SDO Upload35 : xpcethercatlib/EtherCAT Async SDO Upload  index=8193  subIndex=3  sig_type=uint32  sig_dim=1  device_id=0  slave_name=Drive 7 (AKD)  sample_time=1  slave_addr=1006  selected_slave=Term 1 (EK1100)  timeout=500  slave_found=1
      settings: SourceProductName=Simulink Real-Time  SourceProductBaseCode=XP
  EtherCAT Async SDO Upload4 : xpcethercatlib/EtherCAT Async SDO Upload  index=8193  subIndex=2  sig_type=uint32  sig_dim=1  device_id=0  slave_name=Drive 2 (AKD)  sample_time=1  slave_addr=1001  selected_slave=Term 1 (EK1100)  timeout=500  slave_found=1
      settings: SourceProductName=Simulink Real-Time  SourceProductBaseCode=XP
  EtherCAT Async SDO Upload5 : xpcethercatlib/EtherCAT Async SDO Upload  index=8193  subIndex=3  sig_type=uint32  sig_dim=1  device_id=0  slave_name=Drive 1 (AKD)  sample_time=1  slave_addr=1001  selected_slave=Term 1 (EK1100)  timeout=500  slave_found=1
      settings: SourceProductName=Simulink Real-Time  SourceProductBaseCode=XP
  EtherCAT Async SDO Upload6 : xpcethercatlib/EtherCAT Async SDO Upload  index=8192  subIndex=1  sig_type=uint32  sig_dim=1  device_id=0  slave_name=Drive 3 (AKD)  sample_time=1  slave_addr=1002  selected_slave=Term 1 (EK1100)  timeout=500  slave_found=1
      settings: SourceProductName=Simulink Real-Time  SourceProductBaseCode=XP
  EtherCAT Async SDO Upload7 : xpcethercatlib/EtherCAT Async SDO Upload  index=8192  subIndex=2  sig_type=uint32  sig_dim=1  device_id=0  slave_name=Drive 3 (AKD)  sample_time=1  slave_addr=1002  selected_slave=Term 1 (EK1100)  timeout=500  slave_found=1
      settings: SourceProductName=Simulink Real-Time  SourceProductBaseCode=XP
  EtherCAT Async SDO Upload8 : xpcethercatlib/EtherCAT Async SDO Upload  index=8192  subIndex=3  sig_type=uint32  sig_dim=1  device_id=0  slave_name=Drive 3 (AKD)  sample_time=1  slave_addr=1002  selected_slave=Term 1 (EK1100)  timeout=500  slave_found=1
      settings: SourceProductName=Simulink Real-Time  SourceProductBaseCode=XP
  EtherCAT Async SDO Upload9 : xpcethercatlib/EtherCAT Async SDO Upload  index=8193  subIndex=1  sig_type=uint32  sig_dim=1  device_id=0  slave_name=Drive 3 (AKD)  sample_time=1  slave_addr=1002  selected_slave=Term 1 (EK1100)  timeout=500  slave_found=1
      settings: SourceProductName=Simulink Real-Time  SourceProductBaseCode=XP
  Terminator{2..37} (36 alike) : Terminator
  Warnings : Outport
  Errors : Outport  Port=2
  wires:
  EtherCAT Async SDO Upload13/2 -> Terminator15/1
  EtherCAT Async SDO Upload23/2 -> Terminator25/1
  EtherCAT Async SDO Upload25/2 -> Terminator27/1
  EtherCAT Async SDO Upload9/2 -> Terminator11/1
  EtherCAT Async SDO Upload5/2 -> Terminator7/1
  EtherCAT Async SDO Upload30/2 -> Terminator32/1
  EtherCAT Async SDO Upload27/2 -> Terminator29/1
  EtherCAT Async SDO Upload12/2 -> Terminator14/1
  EtherCAT Async SDO Upload24/2 -> Terminator26/1
  EtherCAT Async SDO Upload26/2 -> Terminator28/1
  Bus Creator12/1 -> Bus Creator20/3
  Demux/3 -> EtherCAT Async SDO Upload12/1, EtherCAT Async SDO Upload13/1, EtherCAT Async SDO Upload14/1, EtherCAT Async SDO Upload17/1, EtherCAT Async SDO Upload16/1, EtherCAT Async SDO Upload15/1
  EtherCAT Async SDO Upload30/1 -> Bus Creator18/1
  Demux/2 -> EtherCAT Async SDO Upload11/1, EtherCAT Async SDO Upload10/1, EtherCAT Async SDO Upload9/1, EtherCAT Async SDO Upload6/1, EtherCAT Async SDO Upload7/1, EtherCAT Async SDO Upload8/1
  EtherCAT Async SDO Upload9/1 -> Bus Creator11/1
  EtherCAT Async SDO Upload18/2 -> Terminator20/1
  EtherCAT Async SDO Upload8/2 -> Terminator10/1
  EtherCAT Async SDO Upload11/2 -> Terminator13/1
  Demux/6 -> EtherCAT Async SDO Upload30/1, EtherCAT Async SDO Upload31/1, EtherCAT Async SDO Upload32/1, EtherCAT Async SDO Upload35/1, EtherCAT Async SDO Upload34/1, EtherCAT Async SDO Upload33/1
  Demux/4 -> EtherCAT Async SDO Upload18/1, EtherCAT Async SDO Upload19/1, EtherCAT Async SDO Upload20/1, EtherCAT Async SDO Upload23/1, EtherCAT Async SDO Upload22/1, EtherCAT Async SDO Upload21/1
  EtherCAT Async SDO Upload19/2 -> Terminator21/1
  Bus Creator19/1 -> Bus Creator21/6
  Demux/1 -> EtherCAT Async SDO Upload5/1, EtherCAT Async SDO Upload4/1, EtherCAT Async SDO Upload3/1, EtherCAT Async SDO Upload/1, EtherCAT Async SDO Upload1/1, EtherCAT Async SDO Upload2/1
  EtherCAT Async SDO Upload15/2 -> Terminator17/1
  Bus Creator14/1 -> Bus Creator20/4
  EtherCAT Async SDO Upload34/2 -> Terminator36/1
  Demux/5 -> EtherCAT Async SDO Upload24/1, EtherCAT Async SDO Upload25/1, EtherCAT Async SDO Upload26/1, EtherCAT Async SDO Upload29/1, EtherCAT Async SDO Upload28/1, EtherCAT Async SDO Upload27/1
  EtherCAT Async SDO Upload6/2 -> Terminator8/1
  EtherCAT Async SDO Upload/1 -> Bus Creator1/1
  EtherCAT Async SDO Upload7/2 -> Terminator9/1
  EtherCAT Async SDO Upload16/2 -> Terminator18/1
  Bus Creator13/1 -> Bus Creator21/3
  EtherCAT Async SDO Upload10/2 -> Terminator12/1
  EtherCAT Async SDO Upload35/2 -> Terminator37/1
  EtherCAT Async SDO Upload21/1 -> Bus Creator15/1
  Bus Creator16/1 -> Bus Creator20/5
  EtherCAT Async SDO Upload31/2 -> Terminator33/1
  EtherCAT Async SDO Upload32/1 -> Bus Creator18/3
  EtherCAT Async SDO Upload15/1 -> Bus Creator13/1
  EtherCAT Async SDO Upload/2 -> Terminator2/1
  EtherCAT Async SDO Upload13/1 -> Bus Creator12/2
  EtherCAT Async SDO Upload33/2 -> Terminator35/1
  EtherCAT Async SDO Upload4/2 -> Terminator6/1
  EtherCAT Async SDO Upload28/2 -> Terminator30/1
  EtherCAT Async SDO Upload1/2 -> Terminator3/1
  Bus Creator10/1 -> Bus Creator20/2
  EtherCAT Async SDO Upload8/1 -> Bus Creator10/3
  EtherCAT Async SDO Upload19/1 -> Bus Creator14/2
  EtherCAT Async SDO Upload20/2 -> Terminator22/1
  EtherCAT Async SDO Upload12/1 -> Bus Creator12/1
  EtherCAT Async SDO Upload29/2 -> Terminator31/1
  EtherCAT Async SDO Upload2/1 -> Bus Creator1/3
  EtherCAT Async SDO Upload26/1 -> Bus Creator16/3
  EtherCAT Async SDO Upload22/2 -> Terminator24/1
  EtherCAT Async SDO Upload28/1 -> Bus Creator17/2
  Bus Creator1/1 -> Bus Creator20/1
  EtherCAT Async SDO Upload3/2 -> Terminator5/1
  Bus Creator17/1 -> Bus Creator21/5
  EtherCAT Async SDO Upload2/2 -> Terminator4/1
  EtherCAT Async SDO Upload33/1 -> Bus Creator19/1
  EtherCAT Async SDO Upload17/1 -> Bus Creator13/3
  EtherCAT Async SDO Upload31/1 -> Bus Creator18/2
  EtherCAT Async SDO Upload27/1 -> Bus Creator17/1
  EtherCAT Async SDO Upload1/1 -> Bus Creator1/2
  EtherCAT Async SDO Upload3/1 -> Bus Creator3/1
  EtherCAT Async SDO Upload11/1 -> Bus Creator11/3
  EtherCAT Async SDO Upload7/1 -> Bus Creator10/2
  EtherCAT Async SDO Upload6/1 -> Bus Creator10/1
  EtherCAT Async SDO Upload34/1 -> Bus Creator19/2
  Bus Creator18/1 -> Bus Creator20/6
  EtherCAT Async SDO Upload22/1 -> Bus Creator15/2
  EtherCAT Async SDO Upload23/1 -> Bus Creator15/3
  EtherCAT Async SDO Upload18/1 -> Bus Creator14/1
  EtherCAT Async SDO Upload10/1 -> Bus Creator11/2
  EtherCAT Async SDO Upload14/1 -> Bus Creator12/3
  EtherCAT Async SDO Upload35/1 -> Bus Creator19/3
  EtherCAT Async SDO Upload24/1 -> Bus Creator16/1
  EtherCAT Async SDO Upload20/1 -> Bus Creator14/3
  Bus Creator3/1 -> Bus Creator21/1
  EtherCAT Async SDO Upload4/1 -> Bus Creator3/2
  EtherCAT Async SDO Upload25/1 -> Bus Creator16/2
  EtherCAT Async SDO Upload16/1 -> Bus Creator13/2
  Bus Creator15/1 -> Bus Creator21/4
  Bus Creator11/1 -> Bus Creator21/2
  EtherCAT Async SDO Upload5/1 -> Bus Creator3/3
  EtherCAT Async SDO Upload32/2 -> Terminator34/1
  EtherCAT Async SDO Upload29/1 -> Bus Creator17/3
  EtherCAT Async SDO Upload14/2 -> Terminator16/1
  EtherCAT Async SDO Upload17/2 -> Terminator19/1
  EtherCAT Async SDO Upload21/2 -> Terminator23/1
  Bus Creator21/1 -> Errors/1
  Bus Creator20/1 -> Warnings/1
  Enable/1 -> Demux/1
